simulink model "act2_simulink_sesion3"  (R2020a)
settings: Solver=ode1  StartTime=0.0  StopTime=10.0  FixedStep=1e-3  RelTol=1e-3
undefined symbols (not defined in the file or in its folder): C, R
settings Model: Creator=Jorjolo  LastModifiedBy=spide

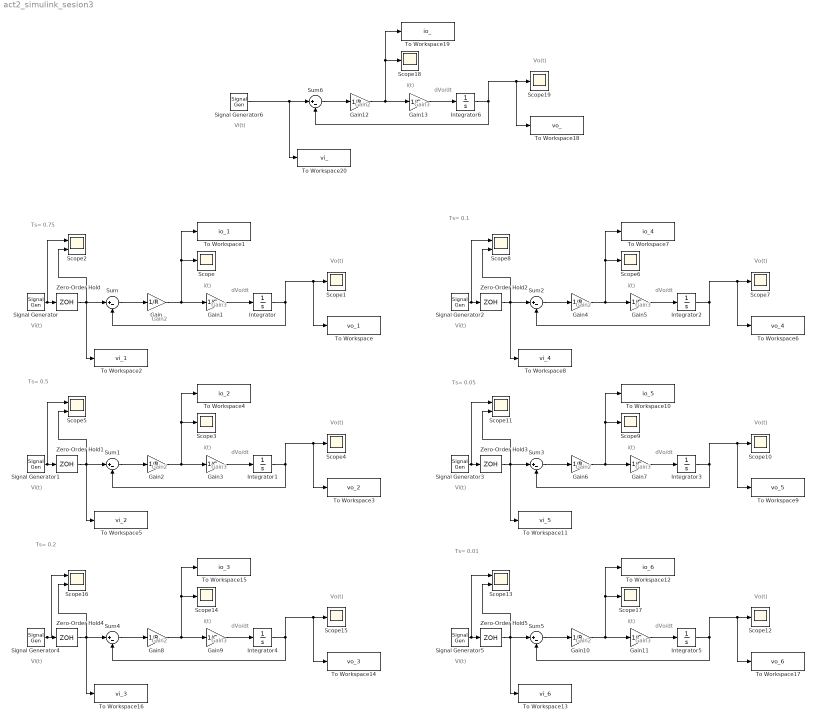
== system act2_simulink_sesion3 ==
  note: Ts= 0.01
  note: Gain3
  note: Gain2
  note: Vi(t)
  note: Vo(t)
  note: dVo/dt
  note: i(t)
  note: i(t)
  note: Vo(t)
  note: Gain3
  note: Vi(t)
  note: Gain2
  note: dVo/dt
  note: Vi(t)
  note: Gain2
  note: dVo/dt
  note: i(t)
  note: Vo(t)
  note: i(t)
  note: Gain3
  note: Gain3
  note: Vo(t)
  note: Gain2
  note: Vi(t)
  note: dVo/dt
  note: Vi(t)
  note: Gain3
  note: Vi(t)
  note: Vo(t)
  note: Gain2
  note: dVo/dt
  note: i(t)
  note: Gain2
  note: Gain3
  note: i(t)
  note: dVo/dt
  note: Vo(t)
  note: Ts= 0.2
  note: Ts= 0.5
  note: Ts= 0.75
  note: Ts= 0.1
  note: Ts= 0.05
  note: Vo(t)
  note: i(t)
  note: Vi(t)
  note: Gain3
  note: dVo/dt
  note: Gain2
  Gain{,2,4,6,8,10,12} (7 alike) : Gain  Gain=1/R
  Gain{1,3,5,7,9,11,13} (7 alike) : Gain  Gain=1/C
  Integrator{,1..6} (7 alike) : Integrator
  Scope{,1,3..4,6..7,9..10,12,14..15,17..19} (14 alike) : Scope
  Scope{2,5,8,11,13,16} (6 alike) : Scope  NumInputPorts=2
  Signal Generator{,1..6} (7 alike) : SignalGenerator  Amplitude=2.5
  Sum{,1..6} (7 alike) : Sum  Inputs=|+-
  To Workspace : ToWorkspace  VariableName=vo_1  SaveFormat=Timeseries  SampleTime=-1
  To Workspace1 : ToWorkspace  VariableName=io_1  SaveFormat=Timeseries  SampleTime=-1
  To Workspace10 : ToWorkspace  VariableName=io_5  SaveFormat=Timeseries  SampleTime=-1
  To Workspace11 : ToWorkspace  VariableName=vi_5  SaveFormat=Timeseries  SampleTime=-1
  To Workspace12 : ToWorkspace  VariableName=io_6  SaveFormat=Timeseries  SampleTime=-1
  To Workspace13 : ToWorkspace  VariableName=vi_6  SaveFormat=Timeseries  SampleTime=-1
  To Workspace14 : ToWorkspace  VariableName=vo_3  SaveFormat=Timeseries  SampleTime=-1
  To Workspace15 : ToWorkspace  VariableName=io_3  SaveFormat=Timeseries  SampleTime=-1
  To Workspace16 : ToWorkspace  VariableName=vi_3  SaveFormat=Timeseries  SampleTime=-1
  To Workspace17 : ToWorkspace  VariableName=vo_6  SaveFormat=Timeseries  SampleTime=-1
  To Workspace18 : ToWorkspace  VariableName=vo_  SaveFormat=Timeseries  SampleTime=-1
  To Workspace19 : ToWorkspace  VariableName=io_  SaveFormat=Timeseries  SampleTime=-1
  To Workspace2 : ToWorkspace  VariableName=vi_1  SaveFormat=Timeseries  SampleTime=-1
  To Workspace20 : ToWorkspace  VariableName=vi_  SaveFormat=Timeseries  SampleTime=-1
  To Workspace3 : ToWorkspace  VariableName=vo_2  SaveFormat=Timeseries  SampleTime=-1
  To Workspace4 : ToWorkspace  VariableName=io_2  SaveFormat=Timeseries  SampleTime=-1
  To Workspace5 : ToWorkspace  VariableName=vi_2  SaveFormat=Timeseries  SampleTime=-1
  To Workspace6 : ToWorkspace  VariableName=vo_4  SaveFormat=Timeseries  SampleTime=-1
  To Workspace7 : ToWorkspace  VariableName=io_4  SaveFormat=Timeseries  SampleTime=-1
  To Workspace8 : ToWorkspace  VariableName=vi_4  SaveFormat=Timeseries  SampleTime=-1
  To Workspace9 : ToWorkspace  VariableName=vo_5  SaveFormat=Timeseries  SampleTime=-1
  Zero-Order Hold : ZeroOrderHold  SampleTime=0.75
  Zero-Order Hold1 : ZeroOrderHold  SampleTime=0.5
  Zero-Order Hold2 : ZeroOrderHold  SampleTime=0.1
  Zero-Order Hold3 : ZeroOrderHold  SampleTime=-1
  Zero-Order Hold4 : ZeroOrderHold  SampleTime=0.2
  Zero-Order Hold5 : ZeroOrderHold  SampleTime=-1
  wires:
  Sum/1 -> Gain/1
  Gain/1 -> To Workspace1/1, Scope/1, Gain1/1
  Gain1/1 -> Integrator/1
  Integrator/1 -> Sum/2, To Workspace/1, Scope1/1
  Signal Generator/1 -> Scope2/1, Zero-Order Hold/1
  Zero-Order Hold/1 -> Scope2/2, To Workspace2/1, Sum/1
  Integrator1/1 -> Sum1/2, To Workspace3/1, Scope4/1
  Zero-Order Hold1/1 -> Scope5/2, To Workspace5/1, Sum1/1
  Gain2/1 -> To Workspace4/1, Scope3/1, Gain3/1
  Sum1/1 -> Gain2/1
  Signal Generator1/1 -> Scope5/1, Zero-Order Hold1/1
  Gain3/1 -> Integrator1/1
  Signal Generator3/1 -> Scope11/1, Zero-Order Hold3/1
  Gain6/1 -> To Workspace10/1, Scope9/1, Gain7/1
  Sum3/1 -> Gain6/1
  Zero-Order Hold3/1 -> Scope11/2, To Workspace11/1, Sum3/1
  Integrator2/1 -> Sum2/2, To Workspace6/1, Scope7/1
  Zero-Order Hold2/1 -> Scope8/2, To Workspace8/1, Sum2/1
  Gain4/1 -> To Workspace7/1, Scope6/1, Gain5/1
  Sum2/1 -> Gain4/1
  Gain7/1 -> Integrator3/1
  Signal Generator2/1 -> Scope8/1, Zero-Order Hold2/1
  Gain5/1 -> Integrator2/1
  Integrator3/1 -> Sum3/2, To Workspace9/1, Scope10/1
  Zero-Order Hold5/1 -> Scope13/2, To Workspace13/1, Sum5/1
  Sum5/1 -> Gain10/1
  Gain10/1 -> To Workspace12/1, Scope17/1, Gain11/1
  Integrator5/1 -> Sum5/2, To Workspace17/1, Scope12/1
  Gain11/1 -> Integrator5/1
  Signal Generator4/1 -> Scope16/1, Zero-Order Hold4/1
  Gain8/1 -> To Workspace15/1, Scope14/1, Gain9/1
  Sum4/1 -> Gain8/1
  Gain9/1 -> Integrator4/1
  Zero-Order Hold4/1 -> Scope16/2, To Workspace16/1, Sum4/1
  Integrator4/1 -> Sum4/2, To Workspace14/1, Scope15/1
  Signal Generator5/1 -> Scope13/1, Zero-Order Hold5/1
  Sum6/1 -> Gain12/1
  Integrator6/1 -> Sum6/2, To Workspace18/1, Scope19/1
  Gain12/1 -> To Workspace19/1, Scope18/1, Gain13/1
  Gain13/1 -> Integrator6/1
  Signal Generator6/1 -> To Workspace20/1, Sum6/1
